simulink model "Ejercicio_20_23_02_17"  (R2013a)
settings: Solver=ode45  StartTime=0.0  StopTime=100  RelTol=1e-3
settings Model: Creator=Miguel  LastModifiedBy=Miguel

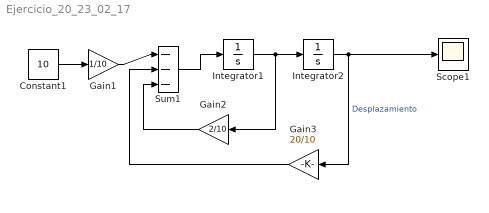
== system Ejercicio_20_23_02_17 ==
  Constant1 : Constant  Value=10
  Gain1 : Gain  Gain=1/10
  Gain2 : Gain  Gain=2/10
  Gain3 : Gain  Gain=20/10
  Integrator1 : Integrator
  Integrator2 : Integrator
  Scope1 : Scope
      settings: ShowLegends=on
  Sum1 : Sum  Inputs=|---
  wires:
  Integrator1/1 -> Gain2/1, Integrator2/1
  Sum1/1 -> Integrator1/1
  Integrator2/1 -> Scope1/1, Gain3/1  "Desplazamiento"
  Gain2/1 -> Sum1/3
  Gain3/1 -> Sum1/2
  Gain1/1 -> Sum1/1
  Constant1/1 -> Gain1/1
